simulink model "sampleModel1791"  (R2023a)
settings: Solver=VariableStepAuto  StartTime=0.0  StopTime=10.0  RelTol=1e-3
libraries: hdlsllib x6, simulink x3
settings Model: Creator=user1  LastModifiedBy=user1

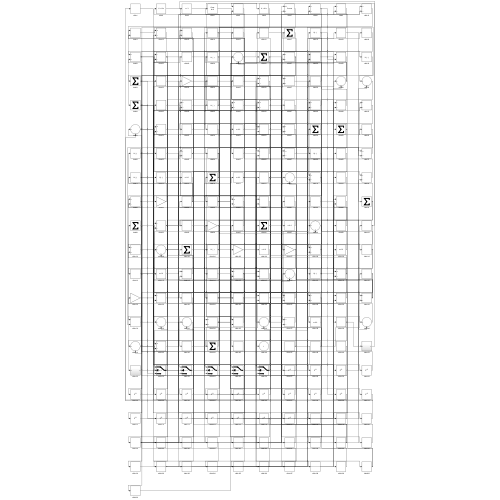
[thumbnail: Simulink's stored preview of the top-level diagram]
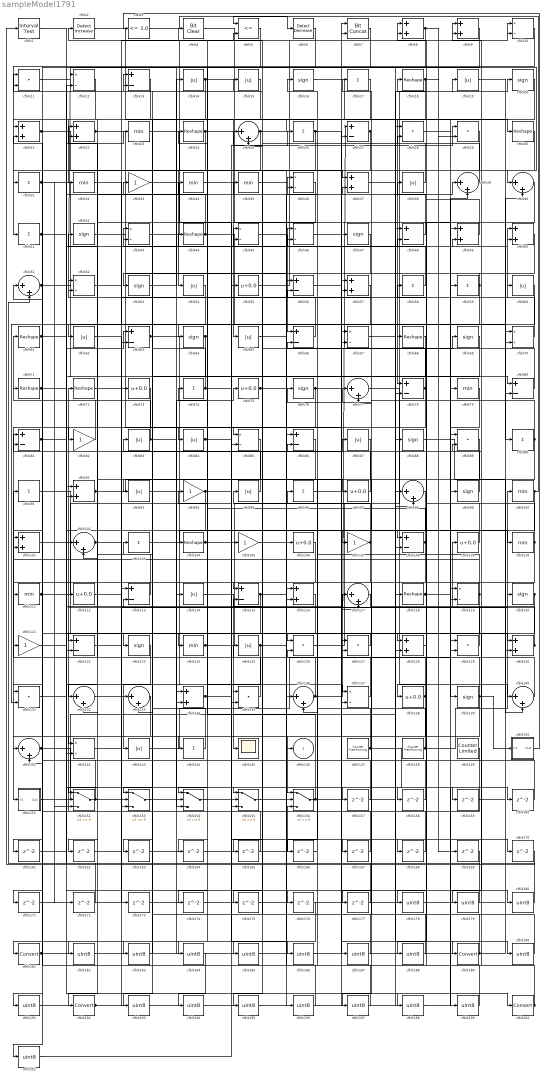
== system sampleModel1791 ==
  cfblk1 : hdlsllib/Logic and Bit Operations/Interval Test  IntervalClosedRight=on  uplimit=0.5  IntervalClosedLeft=on  lowlimit=-0.5  OutDataTypeStr=boolean
  cfblk{10,12,36,43,45..46,52,67,70,85,119,137,142} (13 alike) : Product  Inputs=*/  RndMeth=Zero  SaturateOnIntegerOverflow=on
  cfblk{23,32,34..35,79,100,110..111,124} (9 alike) : MinMax
  cfblk{8..9,21..22,37,49..50,57,92,101,116,128,130,134} (14 alike) : Sum
  cfblk{25,39..40,51,77,98,102,117,132..133,136,140..141} (13 alike) : Sum  Inputs=|++
  cfblk{17,26,31,41,58..59,74,90..91,96,103,144} (12 alike) : Sum  Inputs=+
  cfblk{18,24,30,44,61,68,71..72,104,118} (10 alike) : Reshape
  cfblk{33,82,94,105,107,121} (6 alike) : Gain
  cfblk{55,73,75,97,106,109,112,138} (8 alike) : Bias  Bias=0.0  SaturateOnIntegerOverflow=off
  cfblk{13,27,48,56,63,66,78,80..81,86,108,113,115,122} (14 alike) : Sum  Inputs=+-
  cfblk{11,28..29,89,126..127,129,131,135} (9 alike) : DotProduct  OutDataTypeStr=Inherit: Inherit via internal rule
  cfblk{14..15,19,38,54,60,62,65,83..84,87,93,95,114,125,143} (16 alike) : Abs  SaturateOnIntegerOverflow=off
  cfblk{16,20,42,47,53,64,69,76,88,99,120,123,139} (13 alike) : Signum
  cfblk145 : Scope
  cfblk147 : hdlsllib/Sources/Counter Free-Running  NumBits=16  tsamp=-1
  cfblk148 : hdlsllib/Sources/Counter Free-Running  NumBits=16  tsamp=-1
  cfblk149 : hdlsllib/Sources/Counter Limited  uplimit=7  tsamp=-1
  cfblk150 : Subsystem
      settings: LibrarySourceBlock=|
      | hdlsllib/Ports &
      | Subsystems/Subsystem
  cfblk151 : Subsystem
      settings: LibrarySourceBlock=|
      | hdlsllib/Ports &
      | Subsystems/Subsystem
  cfblk{152..156} (5 alike) : Switch  SaturateOnIntegerOverflow=off  InputSameDT=off
  cfblk{157..177} (21 alike) : Delay  SampleTime=1
  cfblk{178..180,182..188,190..191,193..199,201} (20 alike) : DataTypeConversion  OutDataTypeStr=uint8  SaturateOnIntegerOverflow=off  RndMeth=Floor
  cfblk{181,189,192,200} (4 alike) : DataTypeConversion  SaturateOnIntegerOverflow=off  RndMeth=Floor
  cfblk2 : simulink/Logic and Bit Operations/Detect Increase  vinit=0.0  OutDataTypeStr=boolean
      settings: LibrarySourceBlock=|
      | hdlsllib/Logic and Bit
      | Operations/Detect
      | Increase
  cfblk3 : hdlsllib/Logic and Bit Operations/Compare To Constant  relop=<=  const=3.0  OutDataTypeStr=boolean
  cfblk4 : simulink/Logic and Bit Operations/Bit Clear  iBit=0
      settings: LibrarySourceBlock=|
      | hdlsllib/Logic and Bit
      | Operations/Bit Clear
  cfblk5 : RelationalOperator  Operator=<=  OutDataTypeStr=boolean  InputSameDT=off
  cfblk6 : simulink/Logic and Bit Operations/Detect Decrease  vinit=0.0  OutDataTypeStr=boolean
      settings: LibrarySourceBlock=|
      | hdlsllib/Logic and Bit
      | Operations/Detect
      | Decrease
  cfblk7 : hdlsllib/Logic and Bit Operations/Bit Concat  numInputs=2
  cfblk146 : Outport  VectorParamsAs1DForOutWhenUnconnected=off
  wires:
  cfblk125/1 -> cfblk154/1, cfblk37/2
  cfblk149/1 -> cfblk72/1
  cfblk45/1 -> cfblk66/1
  cfblk110/1 -> cfblk28/2, cfblk131/1, cfblk177/1
  cfblk136/1 -> cfblk27/1, cfblk52/2, cfblk13/2, cfblk25/2
  cfblk36/1 -> cfblk132/1
  cfblk147/1 -> cfblk95/1, cfblk199/1
  cfblk141/1 -> cfblk155/1, cfblk117/1
  cfblk124/1 -> cfblk20/1, cfblk49/2
  cfblk81/1 -> cfblk46/2, cfblk201/1
  cfblk87/1 -> cfblk132/2
  cfblk20/1 -> cfblk123/1
  cfblk63/1 -> cfblk137/1, cfblk43/2
  cfblk16/1 -> cfblk78/1
  cfblk82/1 -> cfblk61/1
  cfblk11/1 -> cfblk40/1
  cfblk10/1 -> cfblk41/1
  cfblk108/1 -> cfblk74/1, cfblk197/1
  cfblk43/1 -> cfblk8/1
  cfblk91/1 -> cfblk126/1
  cfblk67/1 -> cfblk189/1
  cfblk148/1 -> cfblk100/1, cfblk77/1, cfblk43/1
  cfblk54/1 -> cfblk64/1
  cfblk77/1 -> cfblk140/1
  cfblk127/1 -> cfblk122/1
  cfblk130/1 -> cfblk76/1, cfblk112/1, cfblk46/1
  cfblk83/1 -> cfblk71/1, cfblk22/1, cfblk157/1
  cfblk71/1 -> cfblk39/1, cfblk50/2
  cfblk9/1 -> cfblk154/2
  cfblk40/1 -> cfblk138/1
  cfblk151/1(Out1) -> cfblk48/1
  cfblk123/1 -> cfblk143/1
  cfblk22/1 -> cfblk106/1, cfblk62/1
  cfblk64/1 -> cfblk163/1, cfblk164/1
  cfblk55/1 -> cfblk10/1
  cfblk59/1 -> cfblk53/1, cfblk131/2
  cfblk93/1 -> cfblk155/2
  cfblk143/1 -> cfblk79/1
  cfblk17/1 -> cfblk65/1
  cfblk78/1 -> cfblk151/1(In1), cfblk25/1, cfblk162/1
  cfblk38/1 -> cfblk2/1
  cfblk57/1 -> cfblk84/1
  cfblk56/1 -> cfblk47/1
  cfblk129/1 -> cfblk109/1
  cfblk135/1 -> cfblk91/1
  cfblk15/1 -> cfblk142/1
  cfblk44/1 -> cfblk68/1, cfblk22/2
  cfblk31/1 -> cfblk114/1, cfblk152/3
  cfblk48/1 -> cfblk38/1
  cfblk51/1 -> cfblk12/1, cfblk90/1
  cfblk47/1 -> cfblk85/1
  cfblk153/1 -> cfblk75/1
  cfblk24/1 -> cfblk141/1, cfblk56/1
  cfblk39/1 -> cfblk11/1, cfblk11/2
  cfblk134/1 -> cfblk55/1, cfblk186/1
  cfblk144/1 -> cfblk33/1
  cfblk139/1 -> cfblk152/1, cfblk150/1(In1), cfblk126/2
  cfblk131/1 -> cfblk23/1
  cfblk137/1 -> cfblk36/1
  cfblk92/1 -> cfblk97/1, cfblk10/2
  cfblk107/1 -> cfblk122/2, cfblk56/2, cfblk115/1
  cfblk29/1 -> cfblk101/1
  cfblk85/1 -> cfblk124/1
  cfblk25/1 -> cfblk54/1, cfblk30/1
  cfblk117/1 -> cfblk113/2
  cfblk111/1 -> cfblk85/2, cfblk63/1
  cfblk6/1 -> cfblk111/1
  cfblk113/1 -> cfblk81/1
  cfblk95/1 -> cfblk42/1
  cfblk66/1 -> cfblk44/1
  cfblk114/1 -> cfblk145/1
  cfblk99/1 -> cfblk16/1
  cfblk94/1 -> cfblk142/2, cfblk108/1
  cfblk26/1 -> cfblk102/2, cfblk190/1
  cfblk102/1 -> cfblk45/1, cfblk45/2
  cfblk4/1 -> cfblk116/2
  cfblk27/1 -> cfblk92/2, cfblk31/1
  cfblk12/1 -> cfblk21/1
  cfblk14/1 -> cfblk139/1, cfblk32/1
  cfblk2/1 -> cfblk119/1
  cfblk23/1 -> cfblk37/1
  cfblk73/1 -> cfblk82/1
  cfblk100/1 -> cfblk5/1, cfblk155/3
  cfblk41/1 -> cfblk135/1, cfblk153/3, cfblk172/1
  cfblk61/1 -> cfblk141/2, cfblk128/1, cfblk180/1
  cfblk109/1 -> cfblk48/2
  cfblk84/1 -> cfblk26/1, cfblk128/2
  cfblk76/1 -> cfblk154/3, cfblk9/1, cfblk78/2
  cfblk118/1 -> cfblk49/1, cfblk58/1
  cfblk58/1 -> cfblk15/1
  cfblk70/1 -> cfblk50/1
  cfblk53/1 -> cfblk14/1
  cfblk19/1 -> cfblk70/1
  cfblk80/1 -> cfblk17/1
  cfblk138/1 -> cfblk156/1, cfblk115/2
  cfblk119/1 -> cfblk36/2, cfblk101/2, cfblk161/1
  cfblk150/1(Out1) -> cfblk3/1
  cfblk42/1 -> cfblk156/2
  cfblk3/1 -> cfblk6/1
  cfblk79/1 -> cfblk119/2
  cfblk1/1 -> cfblk80/1
  cfblk156/1 -> cfblk28/1, cfblk94/1
  cfblk68/1 -> cfblk93/1
  cfblk120/1 -> cfblk166/1, cfblk179/1
  cfblk33/1 -> cfblk135/2
  cfblk88/1 -> cfblk140/2
  cfblk98/1 -> cfblk192/1
  cfblk112/1 -> cfblk87/1
  cfblk32/1 -> cfblk70/2
  cfblk152/1 -> cfblk51/1, cfblk60/1, cfblk176/1
  cfblk115/1 -> cfblk69/1, cfblk144/1, cfblk175/1
  cfblk126/1 -> cfblk19/1
  cfblk18/1 -> cfblk134/2, cfblk29/2
  cfblk105/1 -> cfblk200/1
  cfblk90/1 -> cfblk146/1, cfblk52/1, cfblk107/1
  cfblk52/1 -> cfblk5/2
  cfblk74/1 -> cfblk13/1, cfblk170/1
  cfblk21/1 -> cfblk102/1, cfblk117/2
  cfblk28/1 -> cfblk59/1
  cfblk8/1 -> cfblk108/2, cfblk169/1
  cfblk140/1 -> cfblk4/1
  cfblk37/1 -> cfblk118/1
  cfblk75/1 -> cfblk127/1, cfblk130/1
  cfblk65/1 -> cfblk136/1
  cfblk49/1 -> cfblk8/2
  cfblk133/1 -> cfblk181/1
  cfblk34/1 -> cfblk57/2
  cfblk142/1 -> cfblk35/1
  cfblk104/1 -> cfblk29/1, cfblk24/1
  cfblk122/1 -> cfblk120/1
  cfblk97/1 -> cfblk34/1
  cfblk103/1 -> cfblk110/1
  cfblk72/1 -> cfblk127/2
  cfblk116/1 -> cfblk153/1
  cfblk157/1 -> cfblk57/1
  cfblk155/1 -> cfblk158/1
  cfblk158/1 -> cfblk92/1
  cfblk132/1 -> cfblk159/1
  cfblk159/1 -> cfblk40/2
  cfblk101/1 -> cfblk160/1
  cfblk160/1 -> cfblk21/2
  cfblk161/1 -> cfblk12/2
  cfblk162/1 -> cfblk153/2
  cfblk163/1 -> cfblk116/1
  cfblk164/1 -> cfblk156/3
  cfblk30/1 -> cfblk165/1
  cfblk165/1 -> cfblk113/1
  cfblk166/1 -> cfblk136/2
  cfblk154/1 -> cfblk167/1
  cfblk167/1 -> cfblk81/2
  cfblk46/1 -> cfblk168/1
  cfblk168/1 -> cfblk66/2
  cfblk169/1 -> cfblk51/2
  cfblk170/1 -> cfblk1/1
  cfblk13/1 -> cfblk171/1
  cfblk171/1 -> cfblk134/1
  cfblk172/1 -> cfblk152/2
  cfblk62/1 -> cfblk173/1
  cfblk173/1 -> cfblk39/2
  cfblk5/1 -> cfblk174/1
  cfblk174/1 -> cfblk80/2
  cfblk175/1 -> cfblk27/2
  cfblk177/1 -> cfblk103/1
  cfblk89/1 -> cfblk178/1
  cfblk178/1 -> cfblk99/1
  cfblk179/1 -> cfblk89/1
  cfblk180/1 -> cfblk89/2
  cfblk181/1 -> cfblk73/1, cfblk130/2, cfblk104/1, cfblk137/2
  cfblk60/1 -> cfblk182/1
  cfblk182/1 -> cfblk133/1
  cfblk106/1 -> cfblk183/1
  cfblk183/1 -> cfblk133/2
  cfblk7/1 -> cfblk184/1
  cfblk69/1 -> cfblk185/1
  cfblk185/1 -> cfblk7/1
  cfblk186/1 -> cfblk7/2
  cfblk96/1 -> cfblk187/1
  cfblk187/1 -> cfblk125/1
  cfblk128/1 -> cfblk188/1
  cfblk188/1 -> cfblk96/1
  cfblk189/1 -> cfblk77/2, cfblk83/1
  cfblk190/1 -> cfblk67/1
  cfblk176/1 -> cfblk191/1
  cfblk191/1 -> cfblk67/2
  cfblk192/1 -> cfblk63/2, cfblk88/1
  cfblk50/1 -> cfblk193/1
  cfblk193/1 -> cfblk98/1
  cfblk184/1 -> cfblk194/1
  cfblk194/1 -> cfblk98/2
  cfblk86/1 -> cfblk195/1
  cfblk195/1 -> cfblk129/2
  cfblk35/1 -> cfblk196/1
  cfblk196/1 -> cfblk86/1
  cfblk197/1 -> cfblk86/2
  cfblk121/1 -> cfblk198/1
  cfblk198/1 -> cfblk129/1
  cfblk199/1 -> cfblk121/1
  cfblk200/1 -> cfblk9/2, cfblk18/1
  cfblk201/1 -> cfblk105/1

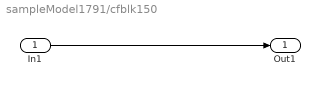
== system sampleModel1791/cfblk150 ==
  In1 : Inport
  Out1 : Outport
  wires:
  In1/1 -> Out1/1

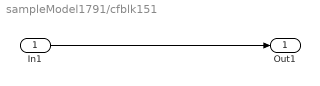
== system sampleModel1791/cfblk151 ==
  In1 : Inport
  Out1 : Outport
  wires:
  In1/1 -> Out1/1
